simulink model "Host_IO_Display"  (R2019b)
settings: Solver=FixedStepAuto  StartTime=0.0  StopTime=inf  FixedStep=TsHost  RelTol=1e-3  EnableMultiTasking=on
InitFcn:
  | host_io_model_init
values from neighbouring files (symbols this model uses):
  FPGAClkRate = DataSampleRate/VectorSamplingFactor    (= 128000000)    [model_init.m]
  S2MM_frame_size = 5e4    (= 50000)    [host_io_model_init.m]    (also in model_init.m = length(signal))
libraries: psp_axi_iio_lib x1
Description:
  | 4x4 IQ ADC/DAC Data capture model for host PC
  | 
  | This model demonstrates capturing data from the FPGA for IQ mixer data. AXI4 register is used
  | to switch between different ADC channels and collect frames of data at every
  | time step of the simulation
  | 
  | The DAC is driven by an NCO. It's frequency is also adjustable from this model as well.
settings Model: Creator=darenlee  LastModifiedBy=tmealey
settings SolverCC: PositivePriorityOrder=on
settings DataIOCC: ReturnWorkspaceOutputs=off
settings OptimizationCC: DefaultParameterBehavior=Inlined  EnhancedBackFolding=on  PassReuseOutputArgsAs=Individual arguments  MaxStackSize=64  OptimizeBlockOrder=speed  DifferentSizesBufferReuse=on  OptimizationCustomize=off  EfficientTunableParamExpr=on
settings DebuggingCC: ParameterTunabilityLossMsg=error  PregeneratedLibrarySubsystemCodeDiagnostic=none  ArithmeticOperatorsInVariantConditions=warning
settings HardwareCC: ProdBitPerPointer=32  ProdBitPerSizeT=32  ProdBitPerPtrDiffT=32  ProdLargestAtomicInteger=Long  ProdLargestAtomicFloat=Double  ProdWordSize=32  ProdLongLongMode=on  ProdHWDeviceType=ARM Compatible->ARM Cortex
settings SFSimCC: SimUseLocalCustomCode=off  MATLABDynamicMemAlloc=off  CustomCodeUndefinedFunction=UseInterfaceOnly
settings RTWCC: SystemTargetFile=ert.tlc  TemplateMakefile=ert_default_tmf  GenerateReport=on  RTWUseLocalCustomCode=off  Toolchain=Linaro AArch32 Linux v6.3.1  IncludeHyperlinkInReport=on  LaunchReport=on  GenerateTraceInfo=on  GenerateTraceReport=on  GenerateTraceReportSl=on  GenerateTraceReportSf=on  GenerateTraceReportEml=on
settings CodeAppCC: ForceParamTrailComments=on  IgnoreCustomStorageClasses=off  OperatorAnnotations=on  SimulinkDataObjDesc=on  SFDataObjDesc=on  InsertBlockDesc=on
settings ERTTargetCC: ERTCustomFileTemplate=example_file_process.tlc

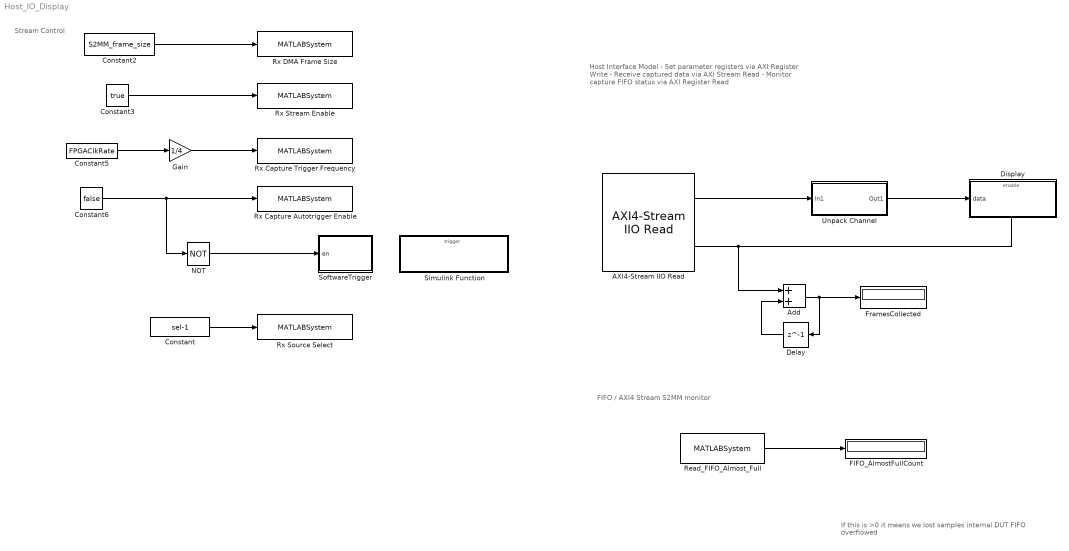
== system Host_IO_Display ==
  note: Host Interface Model
      |
      | - Set parameter registers via AXI Register Write
      | - Receive captured data via AXI Stream Read
      | - Monitor capture FIFO status via AXI Register Read
  note: If this is >0 it means we lost samples
      | internal DUT FIFO overflowed
  note: FIFO / AXI4 Stream S2MM monitor
  note: Stream Control
  AXI4-Stream IIO Read : psp_axi_iio_lib/AXI4-Stream IIO Read  SamplesPerFrame=S2MM_frame_size  DataType=ufix128  Timeout=0  IPAddress=IPAddress  enIO=on  devName=mwipcore0:s2mm0  IPResetMode=none  TLASTMode=auto  TLASTResetMode=never
      settings: SourceProductName=IIO AXI - PSP
  Add : Sum  AccumDataTypeStr=uint32  OutDataTypeStr=uint32
  Constant : Constant  Value=sel-1  OutDataTypeStr=fixdt(0,1,0)  SampleTime=-1  mask{sel=ADC}
      mask prompts: sel "Source select:"
      mask TypeOptions sel: ADC | Pre-DAC
      mask Display: disp(get_param(gcb,'sel'));
  Constant2 : Constant  Value=S2MM_frame_size  OutDataTypeStr=uint32  SampleTime=-1
  Constant3 : Constant  Value=true  SampleTime=-1
  Constant5 : Constant  Value=FPGAClkRate  OutDataTypeStr=uint32  SampleTime=-1
  Constant6 : Constant  Value=false  SampleTime=-1
  Delay : Delay  DelayLength=1
  Display : Subsystem
  FIFO_AlmostFullCount : Display
  FramesCollected : Display
  Gain : Gain  Gain=1/4  OutDataTypeStr=Inherit: Same as input
  NOT : Logic  Operator=NOT  IconShape=distinctive  AllPortsSameDT=off  OutDataTypeStr=boolean
  Read_FIFO_Almost_Full : MATLABSystem  System=pspshared.libiio.aximm.read  DataType=uint32  vectorModeEn=off  outputVectorLength=2  AddressOffsetSrc=Property  AddressOffset=REG_MAP.AXI4_AFIFO_Full  IPAddress=IPAddress  enIO=on  FixedPointDataTypeStr=fixdt(0,14,0)  devName=mwipcore0:mmrd0
      settings: AttributesFormatString=%<AddressOffset>
      mask Type: pspshared.libiio.aximm.read
      mask Display:
      | color('white');
      | plot([100,100,100,100],[100,100,100,100]);
      | plot([0,0,0,0],[0,0,0,0]);
      | color('black');
      | text(50, 48,'AXI4 Register\nIIO Read', 'horizontalAlignment','center','verticalAlignment','middle');
      | color('blue');
      | text(95, 99, 'PSP', 'horizontalAlignment', 'right','verticalAlignment','top');
      | color('black');
      | port_label('output',1, 'Data')
  Rx Capture Autotrigger Enable : MATLABSystem  System=pspshared.libiio.aximm.write  vectorModeEn=off  AddressOffsetSrc=Property  AddressOffset=REG_MAP.rx_auto_trig_en  IPAddress=IPAddress  enIO=on  devName=mwipcore0:mmwr0
      settings: AttributesFormatString=%<AddressOffset>
      mask Type: pspshared.libiio.aximm.write
      mask Display:
      | color('white');
      | plot([100,100,100,100],[100,100,100,100]);
      | plot([0,0,0,0],[0,0,0,0]);
      | color('black');
      | text(50, 48,'AXI4 Register\nIIO Write', 'horizontalAlignment','center','verticalAlignment','middle');
      | color('blue');
      | text(95, 99, 'PSP', 'horizontalAlignment', 'right','verticalAlignment','top');
      | color('black');
      | port_label('input',1, 'Data')
  Rx Capture Trigger Frequency : MATLABSystem  System=pspshared.libiio.aximm.write  vectorModeEn=off  AddressOffsetSrc=Property  AddressOffset=REG_MAP.rx_trigger_freq  IPAddress=IPAddress  enIO=on  devName=mwipcore0:mmwr0
      settings: AttributesFormatString=%<AddressOffset>
      mask Type: pspshared.libiio.aximm.write
      mask Display:
      | color('white');
      | plot([100,100,100,100],[100,100,100,100]);
      | plot([0,0,0,0],[0,0,0,0]);
      | color('black');
      | text(50, 48,'AXI4 Register\nIIO Write', 'horizontalAlignment','center','verticalAlignment','middle');
      | color('blue');
      | text(95, 99, 'PSP', 'horizontalAlignment', 'right','verticalAlignment','top');
      | color('black');
      | port_label('input',1, 'Data')
  Rx DMA Frame Size : MATLABSystem  System=pspshared.libiio.aximm.write  vectorModeEn=off  AddressOffsetSrc=Property  AddressOffset=REG_MAP.rx_frame_size  IPAddress=IPAddress  enIO=on  devName=mwipcore0:mmwr0
      settings: AttributesFormatString=%<AddressOffset>
      mask Type: pspshared.libiio.aximm.write
      mask Display:
      | color('white');
      | plot([100,100,100,100],[100,100,100,100]);
      | plot([0,0,0,0],[0,0,0,0]);
      | color('black');
      | text(50, 48,'AXI4 Register\nIIO Write', 'horizontalAlignment','center','verticalAlignment','middle');
      | color('blue');
      | text(95, 99, 'PSP', 'horizontalAlignment', 'right','verticalAlignment','top');
      | color('black');
      | port_label('input',1, 'Data')
  Rx Source Select : MATLABSystem  System=pspshared.libiio.aximm.write  vectorModeEn=off  AddressOffsetSrc=Property  AddressOffset=REG_MAP.rx_src_select  IPAddress=IPAddress  enIO=on  devName=mwipcore0:mmwr0
      settings: AttributesFormatString=%<AddressOffset>
      mask Type: pspshared.libiio.aximm.write
      mask Display:
      | color('white');
      | plot([100,100,100,100],[100,100,100,100]);
      | plot([0,0,0,0],[0,0,0,0]);
      | color('black');
      | text(50, 48,'AXI4 Register\nIIO Write', 'horizontalAlignment','center','verticalAlignment','middle');
      | color('blue');
      | text(95, 99, 'PSP', 'horizontalAlignment', 'right','verticalAlignment','top');
      | color('black');
      | port_label('input',1, 'Data')
  Rx Stream Enable : MATLABSystem  System=pspshared.libiio.aximm.write  vectorModeEn=off  AddressOffsetSrc=Property  AddressOffset=REG_MAP.rx_stream_en  IPAddress=IPAddress  enIO=on  devName=mwipcore0:mmwr0
      settings: AttributesFormatString=%<AddressOffset>
      mask Type: pspshared.libiio.aximm.write
      mask Display:
      | color('white');
      | plot([100,100,100,100],[100,100,100,100]);
      | plot([0,0,0,0],[0,0,0,0]);
      | color('black');
      | text(50, 48,'AXI4 Register\nIIO Write', 'horizontalAlignment','center','verticalAlignment','middle');
      | color('blue');
      | text(95, 99, 'PSP', 'horizontalAlignment', 'right','verticalAlignment','top');
      | color('black');
      | port_label('input',1, 'Data')
  Simulink Function : Subsystem  TreatAsAtomicUnit=on
      settings: PropExecContextOutsideSubsystem=on
  SoftwareTrigger : MATLAB Function  TreatAsAtomicUnit=on
  Unpack Channel : Subsystem  mask{chan=1}
      mask prompts: chan "Channel:"
      mask TypeOptions chan: 1 | 2 | 3 | 4
      mask Display: fprintf('Channel %d',chan);
  wires:
  Constant2/1 -> Rx DMA Frame Size/1
  Constant3/1 -> Rx Stream Enable/1
  Delay/1 -> Add/2
  Add/1 -> Delay/1, FramesCollected/1
  Constant5/1 -> Gain/1
  Constant6/1 -> NOT/1, Rx Capture Autotrigger Enable/1
  NOT/1 -> SoftwareTrigger/1(en)
  Read_FIFO_Almost_Full/1 -> FIFO_AlmostFullCount/1
  AXI4-Stream IIO Read/1 -> Unpack Channel/1(In1)
  Unpack Channel/1(Out1) -> Display/1(data)
  AXI4-Stream IIO Read/2 -> Add/1, Display/Enable
  Gain/1 -> Rx Capture Trigger Frequency/1
  Constant/1 -> Rx Source Select/1

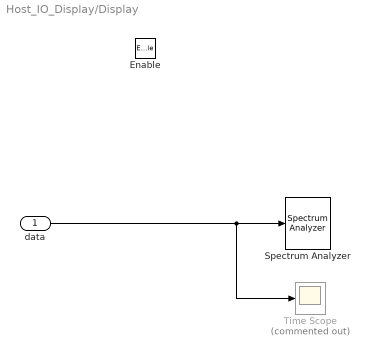
== system Host_IO_Display/Display ==
  data : Inport
  Enable : EnablePort
  Spectrum Analyzer : SpectrumAnalyzer
  Time Scope : Scope  Commented=on
  wires:
  data/1 -> Time Scope/1, Spectrum Analyzer/1

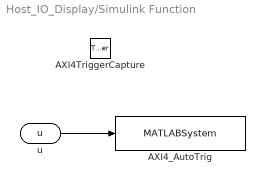
== system Host_IO_Display/Simulink Function ==
  AXI4TriggerCapture : TriggerPort  TriggerType=function-call  IsSimulinkFunction=on  FunctionName=AXI4TriggerCapture  VariantControl=(inherit)
  AXI4_AutoTrig : MATLABSystem  System=pspshared.libiio.aximm.write  vectorModeEn=off  AddressOffsetSrc=Property  AddressOffset=REG_MAP.rx_capture_trig  IPAddress=IPAddress  enIO=on  devName=mwipcore0:mmwr0
      settings: AttributesFormatString=%<AddressOffset>
      mask Type: pspshared.libiio.aximm.write
      mask Display:
      | color('white');
      | plot([100,100,100,100],[100,100,100,100]);
      | plot([0,0,0,0],[0,0,0,0]);
      | color('black');
      | text(50, 48,'AXI4 Register\nIIO Write', 'horizontalAlignment','center','verticalAlignment','middle');
      | color('blue');
      | text(95, 99, 'PSP', 'horizontalAlignment', 'right','verticalAlignment','top');
      | color('black');
      | port_label('input',1, 'Data')
  u : ArgIn  DisableCoverage=on  OutDataTypeStr=boolean  ArgumentName=u
  wires:
  u/1 -> AXI4_AutoTrig/1

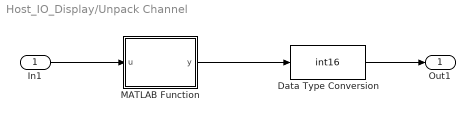
== system Host_IO_Display/Unpack Channel ==
  In1 : Inport
  Data Type Conversion : DataTypeConversion  OutDataTypeStr=int16  ConvertRealWorld=Stored Integer (SI)
  MATLAB Function : MATLAB Function  TreatAsAtomicUnit=on
  Out1 : Outport  VectorParamsAs1DForOutWhenUnconnected=off
  wires:
  MATLAB Function/1(y) -> Data Type Conversion/1
  In1/1 -> MATLAB Function/1(u)
  Data Type Conversion/1 -> Out1/1

== matlab function Host_IO_Display/SoftwareTrigger ==
  data: en input
function TriggerBlk(en)

if en
    AXI4TriggerCapture(true);
    AXI4TriggerCapture(false);
end

end

== matlab function Host_IO_Display/Unpack Channel/MATLAB Function ==
  data: u input; y output; chan parameter
function y = fcn(u, chan)

shiftRe = (chan-1)*32;
shiftIm  = shiftRe+16;
re = uint16(bitsliceget(bitshift(u,-shiftRe), 16,1));
im = uint16(bitsliceget(bitshift(u,-shiftIm), 16,1));

y = complex(re,im);
